simulink model "SCARA"  (R2016a)
settings: Solver=VariableStepAuto  StartTime=0.0  StopTime=10.0  RelTol=1e-3
libraries: powerlib_meascontrol x2, simulink_extras x2
settings Model: Creator=Dominik  LastModifiedBy=Dominik

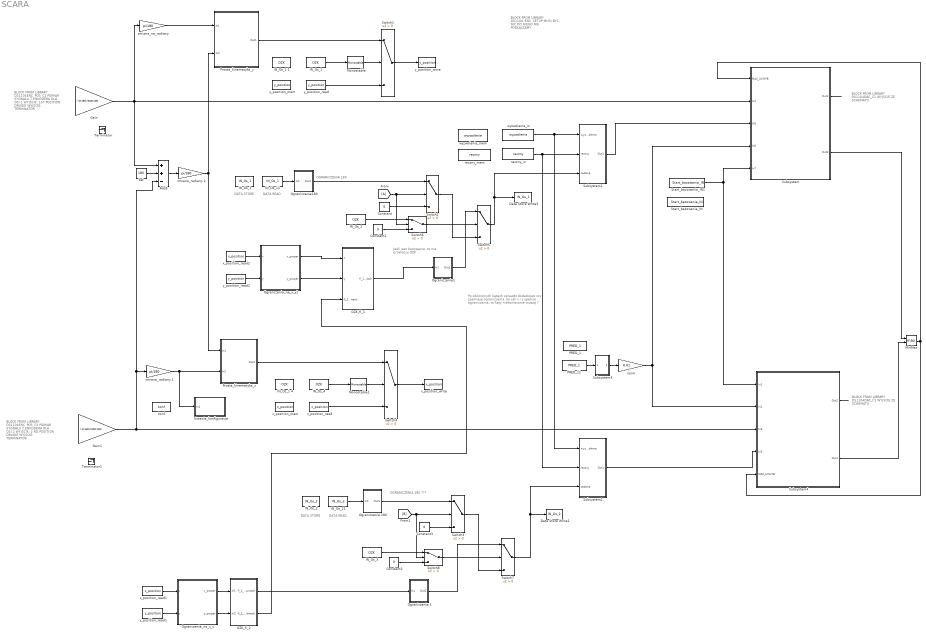
== system SCARA ==
  note: Po obliczonych kątach
      | sprawdź dodatkowo czy spełniają
      | ogranizcenia, bo jak x i y spełnia
      | ograniczenia, to kąty niekoniecznie muszą ?
  note: Jeśli jest bazowanie,
      | to nie przekazuj OZK
  note: DATA READ
  note: DATA STORE
  note: OGRANICZENIA 180
  note: BLOCK FROM LIBRARY
      | DS1104ENC_POS_C1
      | POMIAR SYGNAŁU Z ENKODERA
      | DLA OSI 1
      | WYJŚCIE: 1ST POSITION
      | DRUGIE WYJŚCIE: TERMINATOR
  note: BLOCK FROM LIBRARY
      | DS1104ENC_POS_C2
      | POMIAR SYGNAŁU Z ENKODERA
      | DLA OSI 2
      | WYJŚCIE: 2 ND POSITION
      | DRUGIE WYJŚCIE: TERMINATOR
  note: BLOCK FROM LIBRARY
      | DS1104_ENC_SETUP
      | MUSI BYĆ, NIC DO NIEGO
      | NIE PODŁĄCZAMY
  note: BLOCK FROM LIBRARY
      | DS1104DAC_C1
      | WYJŚCIE ZE SCHEMATU
  note: BLOCK FROM LIBRARY
      | DS1104DAC_C1
      | WYJŚCIE ZE SCHEMATU
  note: OGRANICZENIA 180 ???
  note: DATA STORE
  note: DATA READ
  Add5 : Sum  Inputs=++-
  Constant{,1..3} (4 alike) : Constant  Value=0
  Data Store Write1 : DataStoreWrite  DataStoreName=IN_Os_2
  Data Store Write3 : DataStoreWrite  DataStoreName=IN_Os_1
  Gain : Gain  Gain=(-2*180)/(500*128)
  Gain1 : Gain  Gain=(-2*180)/(500*128)
  IN_Os_{1..4} (4 alike) : DataStoreRead  DataStoreName=OZK
  "IN_Os_1 " : DataStoreMemory  DataStoreName=IN_Os_1  ReadBeforeWriteMsg=warning  WriteAfterWriteMsg=warning  WriteAfterReadMsg=warning  ShowAdditionalParam=off
  IN_Os_1 1 : DataStoreMemory  DataStoreName=OZK  ReadBeforeWriteMsg=warning  WriteAfterWriteMsg=warning  WriteAfterReadMsg=warning  ShowAdditionalParam=off
  IN_Os_1 4 : DataStoreMemory  DataStoreName=OZK  ReadBeforeWriteMsg=warning  WriteAfterWriteMsg=warning  WriteAfterReadMsg=warning  ShowAdditionalParam=off
  IN_Os_11 : DataStoreRead  DataStoreName=IN_Os_1
  "IN_Os_2 " : DataStoreMemory  DataStoreName=IN_Os_2  ReadBeforeWriteMsg=warning  WriteAfterWriteMsg=warning  WriteAfterReadMsg=warning  ShowAdditionalParam=off
  IN_Os_21 : DataStoreRead  DataStoreName=IN_Os_2
  MinMax : MinMax  Function=max  Inputs=2
  Monostable : powerlib_meascontrol/Logic/Monostable  EdgeDetect=Rising  PulseDuration=0.015  ic=0  Ts=0
  Monostable1 : powerlib_meascontrol/Logic/Monostable  EdgeDetect=Rising  PulseDuration=0.015  ic=0  Ts=0
  OZK_fi_1 : Subsystem
  OZK_fi_2 : Subsystem
  Ogranczenia_na_x_y : Subsystem
  Ogranczenia_na_x_y1 : Subsystem
  Ograniczenia 1 : Subsystem
  Ograniczenia 180 : Subsystem
  Ograniczenie1 : Subsystem
  Ograniczenie180 : Subsystem
  "PRED_1 " : DataStoreMemory  DataStoreName=PRED_1  ReadBeforeWriteMsg=warning  WriteAfterWriteMsg=warning  WriteAfterReadMsg=warning  InitialValue=50  ShowAdditionalParam=off
  "PRED_11 " : DataStoreRead  DataStoreName=PRED_1
  Prosta_kinematyka_x : Subsystem
  Prosta_kinematyka_y : Subsystem
  "Start_bazowania_IN " : DataStoreMemory  DataStoreName=Start_bazowania_IN  ReadBeforeWriteMsg=warning  WriteAfterWriteMsg=warning  WriteAfterReadMsg=warning  ShowAdditionalParam=off
  Start_bazowania_IN1 : DataStoreRead  DataStoreName=Start_bazowania_IN
  Subsystem : Subsystem
  Subsystem1 : Subsystem
  Subsystem2 : Subsystem
  Subsystem3 : Subsystem
  Subsystem4 : Subsystem
  Switch{1..8} (8 alike) : Switch  Criteria=u2 > Threshold
  Terminator : Terminator
  Terminator1 : Terminator
  Ustawia_konfiguracje : Subsystem
  "kat " : Constant  Value=180
  konf : DataStoreMemory  DataStoreName=konf  ReadBeforeWriteMsg=warning  WriteAfterWriteMsg=warning  WriteAfterReadMsg=warning  ShowAdditionalParam=off
  norm : Gain  Gain=0.01
  "reczny_in " : DataStoreRead  DataStoreName=reczny
  reczny_mem : DataStoreMemory  DataStoreName=reczny  ReadBeforeWriteMsg=warning  WriteAfterWriteMsg=warning  WriteAfterReadMsg=warning  ShowAdditionalParam=off
  "wyzwolenie_in " : DataStoreRead  DataStoreName=wyzwolenie
  wyzwolenie_mem : DataStoreMemory  DataStoreName=wyzwolenie  ReadBeforeWriteMsg=warning  WriteAfterWriteMsg=warning  WriteAfterReadMsg=warning  ShowAdditionalParam=off
  x_position_mem : DataStoreMemory  DataStoreName=x_position  ReadBeforeWriteMsg=warning  WriteAfterWriteMsg=warning  WriteAfterReadMsg=warning  ShowAdditionalParam=off
  x_position_read : DataStoreRead  DataStoreName=x_position
  x_position_read1 : DataStoreRead  DataStoreName=x_position
  x_position_read2 : DataStoreRead  DataStoreName=x_position
  x_position_write : DataStoreWrite  DataStoreName=x_position
  "y_position_mem " : DataStoreMemory  DataStoreName=y_position  ReadBeforeWriteMsg=warning  WriteAfterWriteMsg=warning  WriteAfterReadMsg=warning  ShowAdditionalParam=off
  y_position_read : DataStoreRead  DataStoreName=y_position
  y_position_read1 : DataStoreRead  DataStoreName=y_position
  y_position_read2 : DataStoreRead  DataStoreName=y_position
  y_position_write : DataStoreWrite  DataStoreName=y_position
  "zmiana_na_radiany " : Gain  Gain=pi/180
  zmiana_radiany 1 : Gain  Gain=pi/180
  zmiana_radiany 2 : Gain  Gain=pi/180
  wires:
  ? -> Gain/1
  ? -> Gain1/1
  ? -> Terminator/1
  ? -> Terminator1/1
  IN_Os_11/1 -> Ograniczenie180/1(In1)
  IN_Os_21/1 -> Ograniczenia 180/1(In1)
  Start_bazowania_IN1/1 -> Subsystem/5(In7), Subsystem4/1(In1)
  Constant/1 -> Switch2/3
  Ograniczenie180/1(Out1) -> Switch2/1
  [A] -> Switch6/2, Switch2/2
  Ograniczenia 180/1(Out1) -> Switch3/1
  Constant3/1 -> Switch3/3
  "wyzwolenie_in "/1 -> Subsystem1/1(wyzwolenie), Subsystem2/1(wyzwolenie)
  "reczny_in "/1 -> Subsystem1/2("reczny "), Subsystem2/2("reczny ")
  "PRED_11 "/1 -> Subsystem3/1(In2)
  norm/1 -> Subsystem4/2(In2), Subsystem/4(In6)
  Subsystem3/1(Out1) -> norm/1
  Subsystem1/1(Out1) -> Subsystem/3(In5)
  Subsystem/1(Out1) -> ?
  Gain1/1 -> Add5/3, zmiana_radiany 1/1, Subsystem4/3(In3)
  Subsystem2/1(Out1) -> Subsystem4/4(In5)
  Subsystem4/1(Out2) -> ?
  Subsystem/2(Out2) -> MinMax/1
  Subsystem4/2(Out1) -> MinMax/2
  MinMax/1 -> Subsystem4/5("MAX_UCHYB "), Subsystem/1("MAX_UCHYB ")
  IN_Os_1/1 -> Monostable/1
  y_position_read/1 -> Switch1/3
  Monostable/1 -> Switch1/2
  Switch1/1 -> y_position_write/1
  IN_Os_4/1 -> Monostable1/1
  x_position_read/1 -> Switch4/3
  Monostable1/1 -> Switch4/2
  Switch4/1 -> x_position_write/1
  "kat "/1 -> Add5/2
  Gain/1 -> "zmiana_na_radiany "/1, Add5/1, Subsystem/2(In2)
  Add5/1 -> zmiana_radiany 2/1
  zmiana_radiany 2/1 -> Prosta_kinematyka_y/2(In2), Prosta_kinematyka_x/1(In1)
  zmiana_radiany 1/1 -> Ustawia_konfiguracje/1(In1), Prosta_kinematyka_x/2(In2)
  Prosta_kinematyka_x/1(Out1) -> Switch4/1
  "zmiana_na_radiany "/1 -> Prosta_kinematyka_y/1(In1)
  Prosta_kinematyka_y/1(Out1) -> Switch1/1
  x_position_read1/1 -> Ogranczenia_na_x_y/1(x)
  y_position_read1/1 -> Ogranczenia_na_x_y/2(y)
  Switch5/1 -> Data Store Write3/1, Subsystem1/3("zadana ")
  Switch2/1 -> Switch5/3
  Ograniczenie1/1(Out1) -> Switch5/1
  IN_Os_2/1 -> Switch6/1
  Constant1/1 -> Switch6/3
  Switch6/1 -> Switch5/2
  x_position_read2/1 -> Ogranczenia_na_x_y1/1(x)
  y_position_read2/1 -> Ogranczenia_na_x_y1/2(y)
  Ogranczenia_na_x_y/1(x_proper) -> OZK_fi_2/1(In1)
  Ogranczenia_na_x_y/2(y_proper) -> OZK_fi_2/2(In2)
  OZK_fi_2/1(fi_2_w_stopniach) -> Ograniczenia 1/1(In1)
  [B] -> Switch8/2, Switch3/2
  IN_Os_3/1 -> Switch8/1
  Constant2/1 -> Switch8/3
  Switch3/1 -> Switch7/3
  Switch8/1 -> Switch7/2
  Ograniczenia 1/1(Out1) -> Switch7/1
  Switch7/1 -> Subsystem2/3("zadana "), Data Store Write1/1
  OZK_fi_2/2(fi_2_w_radianach) -> OZK_fi_1/3(fi_2_w_radianach)
  Ogranczenia_na_x_y1/1(x_proper) -> OZK_fi_1/1(x)
  Ogranczenia_na_x_y1/2(y_proper) -> OZK_fi_1/2(y)
  OZK_fi_1/1(fi_1_w_stopniach) -> Ograniczenie1/1(In1)

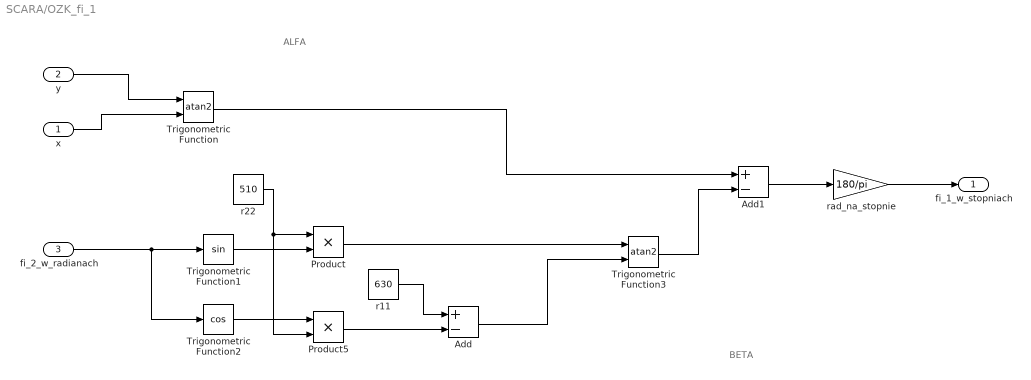
== system SCARA/OZK_fi_1 ==
  note: BETA
  note: ALFA
  x : Inport
  y : Inport  Port=2
  fi_2_w_radianach : Inport  Port=3
  Add : Sum  Inputs=+-
  Add1 : Sum  Inputs=+-
  Product : Product
  Product5 : Product
  Trigonometric Function : Trigonometry  Operator=atan2
  Trigonometric Function1 : Trigonometry
  Trigonometric Function2 : Trigonometry  Operator=cos
  Trigonometric Function3 : Trigonometry  Operator=atan2
  r11 : Constant  Value=630
  r22 : Constant  Value=510
  rad_na_stopnie : Gain  Gain=180/pi
  fi_1_w_stopniach : Outport
  wires:
  fi_2_w_radianach/1 -> Trigonometric Function2/1, Trigonometric Function1/1
  Trigonometric Function1/1 -> Product/2
  r22/1 -> Product5/2, Product/1
  Product/1 -> Trigonometric Function3/1
  Trigonometric Function2/1 -> Product5/1
  r11/1 -> Add/1
  Product5/1 -> Add/2
  Add/1 -> Trigonometric Function3/2
  y/1 -> Trigonometric Function/1
  x/1 -> Trigonometric Function/2
  Trigonometric Function/1 -> Add1/1
  Trigonometric Function3/1 -> Add1/2
  Add1/1 -> rad_na_stopnie/1
  rad_na_stopnie/1 -> fi_1_w_stopniach/1

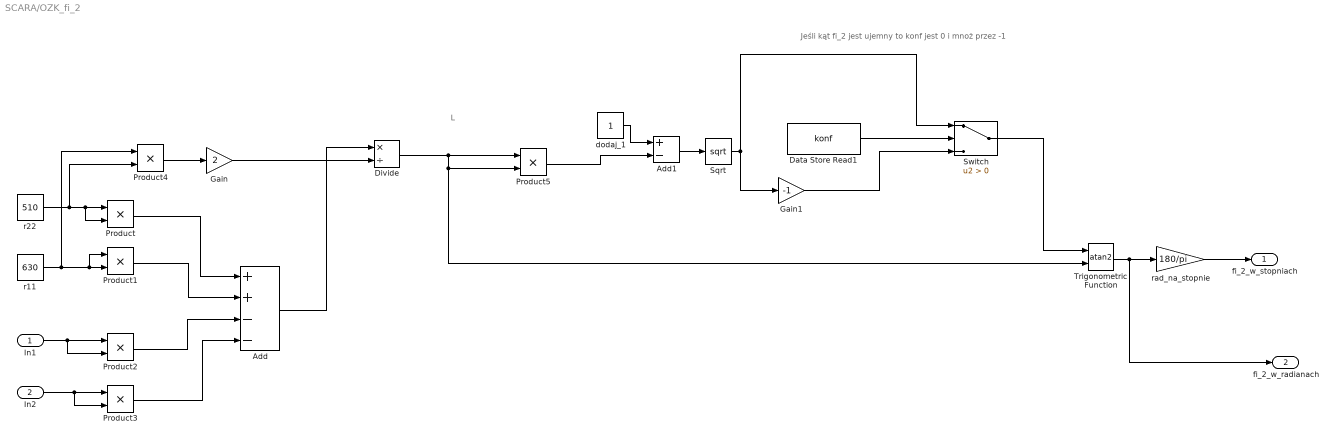
== system SCARA/OZK_fi_2 ==
  note: L
  note: Jeśli kąt fi_2 jest ujemny to konf jest 0
      | i mnoż przez -1
  In1 : Inport
  In2 : Inport  Port=2
  Add : Sum  Inputs=++--
  Add1 : Sum  Inputs=+-
  Data Store Read1 : DataStoreRead  DataStoreName=konf
  Divide : Product  Inputs=*/
  Gain : Gain  Gain=2
  Gain1 : Gain  Gain=-1
  Product{,1..5} (6 alike) : Product
  Sqrt : Sqrt  SaturateOnIntegerOverflow=on
  Switch : Switch  Criteria=u2 > Threshold
  Trigonometric Function : Trigonometry  Operator=atan2
  dodaj_1 : Constant
  r11 : Constant  Value=630
  r22 : Constant  Value=510
  rad_na_stopnie : Gain  Gain=180/pi
  fi_2_w_stopniach : Outport
  fi_2_w_radianach : Outport  Port=2
  wires:
  r22/1 -> Product/2, Product/1, Product4/2
  In1/1 -> Product2/2, Product2/1
  Product1/1 -> Add/2
  Product3/1 -> Add/4
  In2/1 -> Product3/2, Product3/1
  Product/1 -> Add/1
  Product2/1 -> Add/3
  r11/1 -> Product1/1, Product1/2, Product4/1
  Add/1 -> Divide/1
  Product4/1 -> Gain/1
  Gain/1 -> Divide/2
  dodaj_1/1 -> Add1/1
  Add1/1 -> Sqrt/1
  Sqrt/1 -> Gain1/1, Switch/1
  Gain1/1 -> Switch/3
  Switch/1 -> Trigonometric Function/1
  Trigonometric Function/1 -> fi_2_w_radianach/1, rad_na_stopnie/1
  Product5/1 -> Add1/2
  Divide/1 -> Trigonometric Function/2, Product5/2, Product5/1
  Data Store Read1/1 -> Switch/2
  rad_na_stopnie/1 -> fi_2_w_stopniach/1

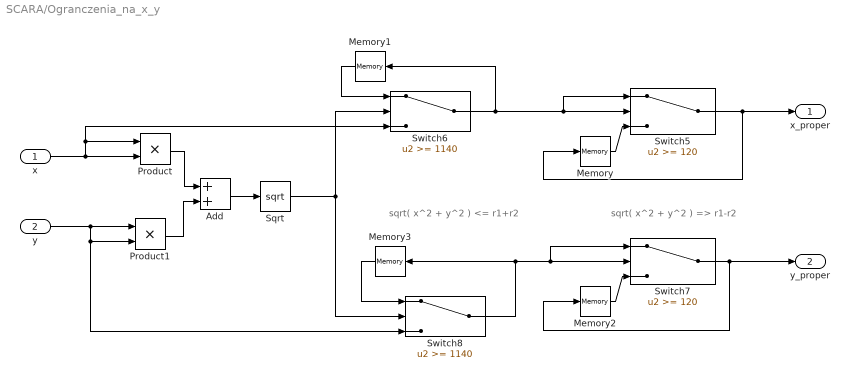
== system SCARA/Ogranczenia_na_x_y ==
  note: sqrt( x^2 + y^2 ) <= r1+r2
  note: sqrt( x^2 + y^2 ) => r1-r2
  x : Inport
  y : Inport  Port=2
  Add : Sum
  Memory{,1..3} (4 alike) : Memory
  Product : Product
  Product1 : Product
  Sqrt : Sqrt  SaturateOnIntegerOverflow=on
  Switch5 : Switch  Threshold=120
  Switch6 : Switch  Threshold=1140
  Switch7 : Switch  Threshold=120
  Switch8 : Switch  Threshold=1140
  x_proper : Outport
  y_proper : Outport  Port=2
  wires:
  Switch5/1 -> x_proper/1, Memory/1
  Switch6/1 -> Switch5/1, Switch5/2, Memory1/1
  Product1/1 -> Add/2
  Memory1/1 -> Switch6/1
  Memory/1 -> Switch5/3
  Switch7/1 -> y_proper/1, Memory2/1
  Memory2/1 -> Switch7/3
  Memory3/1 -> Switch8/1
  Sqrt/1 -> Switch8/2, Switch6/2
  Switch8/1 -> Switch7/1, Switch7/2, Memory3/1
  Add/1 -> Sqrt/1
  y/1 -> Switch8/3, Product1/2, Product1/1
  x/1 -> Product/2, Switch6/3, Product/1
  Product/1 -> Add/1

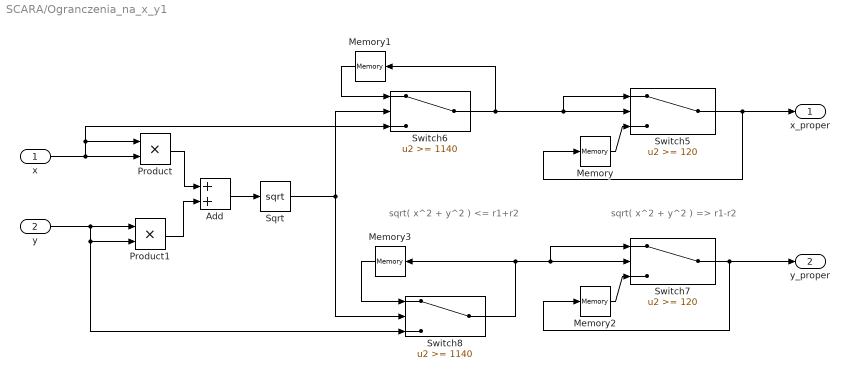
== system SCARA/Ogranczenia_na_x_y1 ==
  note: sqrt( x^2 + y^2 ) <= r1+r2
  note: sqrt( x^2 + y^2 ) => r1-r2
  x : Inport
  y : Inport  Port=2
  Add : Sum
  Memory{,1..3} (4 alike) : Memory
  Product : Product
  Product1 : Product
  Sqrt : Sqrt  SaturateOnIntegerOverflow=on
  Switch5 : Switch  Threshold=120
  Switch6 : Switch  Threshold=1140
  Switch7 : Switch  Threshold=120
  Switch8 : Switch  Threshold=1140
  x_proper : Outport
  y_proper : Outport  Port=2
  wires:
  Switch5/1 -> x_proper/1, Memory/1
  Switch6/1 -> Switch5/1, Switch5/2, Memory1/1
  Product1/1 -> Add/2
  Memory1/1 -> Switch6/1
  Memory/1 -> Switch5/3
  Switch7/1 -> y_proper/1, Memory2/1
  Memory2/1 -> Switch7/3
  Memory3/1 -> Switch8/1
  Sqrt/1 -> Switch8/2, Switch6/2
  Switch8/1 -> Switch7/1, Switch7/2, Memory3/1
  Add/1 -> Sqrt/1
  y/1 -> Switch8/3, Product1/2, Product1/1
  x/1 -> Product/2, Switch6/3, Product/1
  Product/1 -> Add/1

== system SCARA/Ograniczenia 1 ==
  In1 : Inport
  Abs : Abs
  Memory : Memory
  Switch : Switch  Criteria=u2 > Threshold  Threshold=40
  Out1 : Outport
  wires:
  In1/1 -> Switch/3, Abs/1
  Abs/1 -> Switch/2
  Switch/1 -> Memory/1, Out1/1
  Memory/1 -> Switch/1

== system SCARA/Ograniczenia 180 ==
  In1 : Inport
  Abs : Abs
  Memory : Memory
  Switch : Switch  Criteria=u2 > Threshold  Threshold=40
  Out1 : Outport
  wires:
  In1/1 -> Switch/3, Abs/1
  Abs/1 -> Switch/2
  Switch/1 -> Memory/1, Out1/1
  Memory/1 -> Switch/1

== system SCARA/Ograniczenie1 ==
  In1 : Inport
  Abs : Abs
  Memory : Memory
  Switch : Switch  Criteria=u2 > Threshold  Threshold=180
  Out1 : Outport
  wires:
  In1/1 -> Switch/3, Abs/1
  Abs/1 -> Switch/2
  Switch/1 -> Memory/1, Out1/1
  Memory/1 -> Switch/1

== system SCARA/Ograniczenie180 ==
  In1 : Inport
  Abs : Abs
  Memory : Memory
  Switch : Switch  Criteria=u2 > Threshold  Threshold=180
  Out1 : Outport
  wires:
  In1/1 -> Switch/3, Abs/1
  Abs/1 -> Switch/2
  Switch/1 -> Memory/1, Out1/1
  Memory/1 -> Switch/1

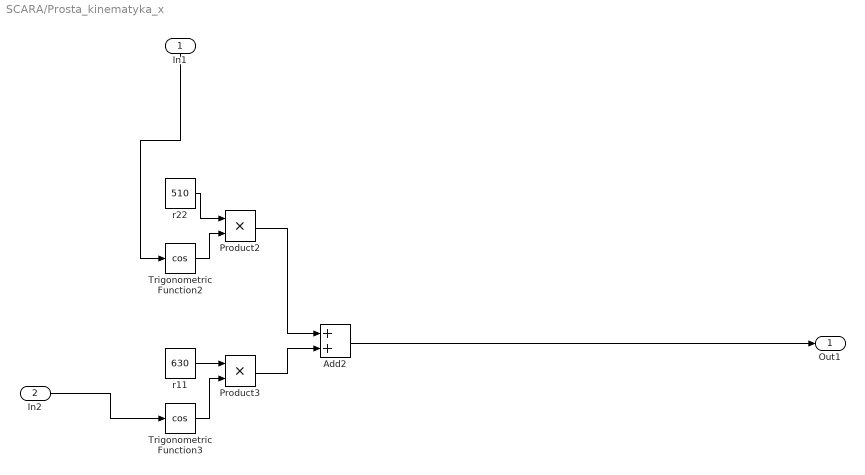
== system SCARA/Prosta_kinematyka_x ==
  In1 : Inport
  In2 : Inport  Port=2
  Add2 : Sum
  Product2 : Product
  Product3 : Product
  Trigonometric Function2 : Trigonometry  Operator=cos
  Trigonometric Function3 : Trigonometry  Operator=cos
  r11 : Constant  Value=630
  r22 : Constant  Value=510
  Out1 : Outport
  wires:
  In2/1 -> Trigonometric Function3/1
  r11/1 -> Product3/1
  r22/1 -> Product2/1
  Add2/1 -> Out1/1
  Trigonometric Function2/1 -> Product2/2
  Trigonometric Function3/1 -> Product3/2
  Product2/1 -> Add2/1
  Product3/1 -> Add2/2
  In1/1 -> Trigonometric Function2/1

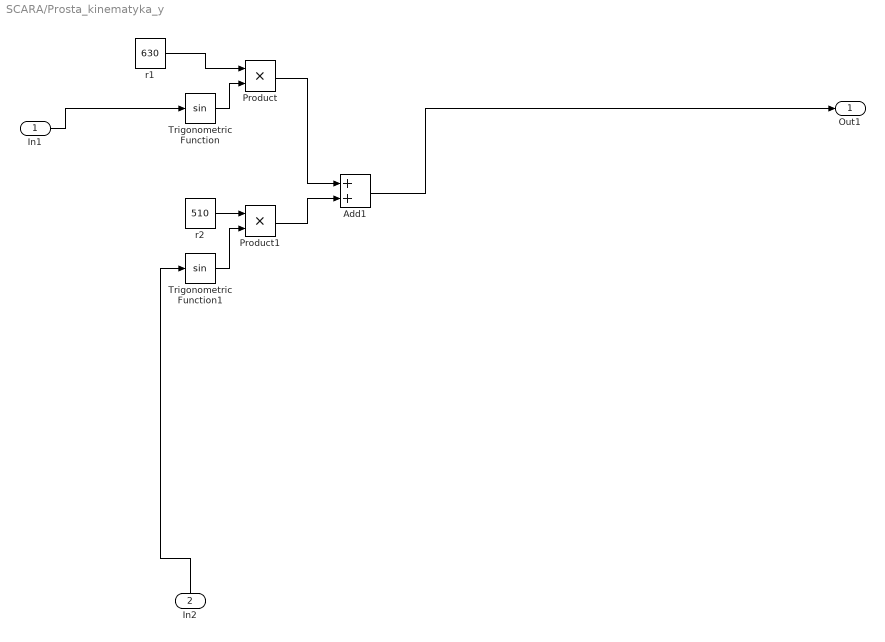
== system SCARA/Prosta_kinematyka_y ==
  In1 : Inport
  In2 : Inport  Port=2
  Add1 : Sum
  Product : Product
  Product1 : Product
  Trigonometric Function : Trigonometry
  Trigonometric Function1 : Trigonometry
  r1 : Constant  Value=630
  r2 : Constant  Value=510
  Out1 : Outport
  wires:
  In1/1 -> Trigonometric Function/1
  Add1/1 -> Out1/1
  r1/1 -> Product/1
  Product/1 -> Add1/1
  Trigonometric Function/1 -> Product/2
  Trigonometric Function1/1 -> Product1/2
  Product1/1 -> Add1/2
  In2/1 -> Trigonometric Function1/1
  r2/1 -> Product1/1

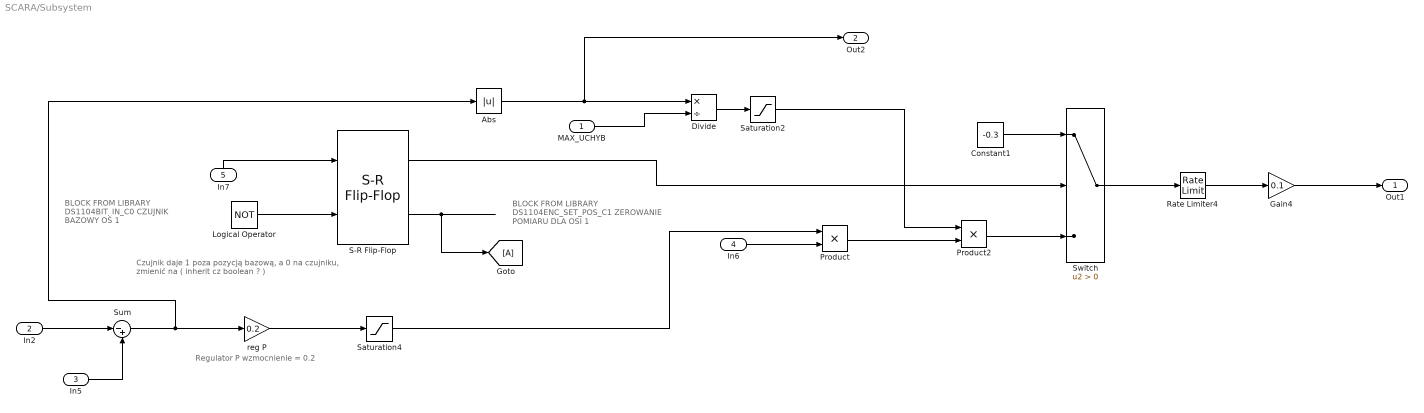
== system SCARA/Subsystem ==
  note: Czujnik daje 1 poza pozycją bazową,
      | a 0 na czujniku, zmienić na ( inherit cz boolean ? )
  note: Regulator P wzmocnienie = 0.2
  note: BLOCK FROM LIBRARY
      | DS1104BIT_IN_C0
      | CZUJNIK BAZOWY OŚ 1
  note: BLOCK FROM LIBRARY
      | DS1104ENC_SET_POS_C1
      | ZEROWANIE POMIARU DLA OSI 1
  "MAX_UCHYB " : Inport
  In2 : Inport  Port=2
  In5 : Inport  Port=3
  In6 : Inport  Port=4
  In7 : Inport  Port=5
  Abs : Abs
  Constant1 : Constant  Value=-0.3
  Divide : Product  Inputs=*/
  Gain4 : Gain  Gain=0.1
  Logical Operator : Logic  Operator=NOT  AllPortsSameDT=off
  Product : Product
  Product2 : Product
  Rate Limiter4 : RateLimiter  RisingSlewLimit=50  FallingSlewLimit=-50  SampleTimeMode=inherited
  S-R Flip-Flop : simulink_extras/Flip Flops/S-R Flip-Flop  initial_condition=0
  Saturation2 : Saturate  UpperLimit=1  LowerLimit=0.001
  Saturation4 : Saturate  UpperLimit=3  LowerLimit=-3
  Sum : Sum  Inputs=|-+
  Switch : Switch  Criteria=u2 > Threshold
  reg P : Gain  Gain=0.2
  Out1 : Outport
  Out2 : Outport  Port=2
  wires:
  Sum/1 -> reg P/1, Abs/1
  Abs/1 -> Out2/1, Divide/1
  "MAX_UCHYB "/1 -> Divide/2
  Divide/1 -> Saturation2/1
  Product/1 -> Product2/2
  Saturation2/1 -> Product2/1
  In7/1 -> S-R Flip-Flop/1
  In6/1 -> Product/2
  In2/1 -> Sum/1
  Rate Limiter4/1 -> Gain4/1
  reg P/1 -> Saturation4/1
  Gain4/1 -> Out1/1
  S-R Flip-Flop/2 -> [A]
  Logical Operator/1 -> S-R Flip-Flop/2
  Switch/1 -> Rate Limiter4/1
  Constant1/1 -> Switch/1
  S-R Flip-Flop/1 -> Switch/2
  ? -> Logical Operator/1
  In5/1 -> Sum/2
  Saturation4/1 -> Product/1
  Product2/1 -> Switch/3

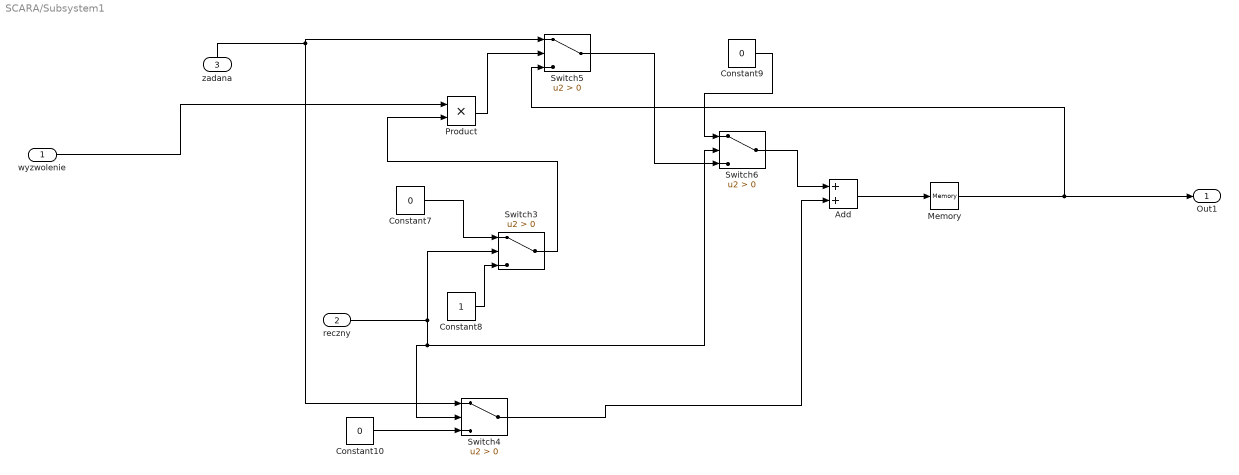
== system SCARA/Subsystem1 ==
  wyzwolenie : Inport
  "reczny " : Inport  Port=2
  "zadana " : Inport  Port=3
  Add : Sum
  Constant10 : Constant  Value=0
  Constant7 : Constant  Value=0
  Constant8 : Constant
  Constant9 : Constant  Value=0
  Memory : Memory
  Product : Product
  Switch{3..6} (4 alike) : Switch  Criteria=u2 > Threshold
  Out1 : Outport
  wires:
  Constant7/1 -> Switch3/1
  Switch4/1 -> Add/2
  "reczny "/1 -> Switch3/2, Switch4/2, Switch6/2
  wyzwolenie/1 -> Product/1
  Add/1 -> Memory/1
  Product/1 -> Switch5/2
  Switch5/1 -> Switch6/3
  "zadana "/1 -> Switch4/1, Switch5/1
  Memory/1 -> Out1/1, Switch5/3
  Constant8/1 -> Switch3/3
  Constant9/1 -> Switch6/1
  Constant10/1 -> Switch4/3
  Switch3/1 -> Product/2
  Switch6/1 -> Add/1

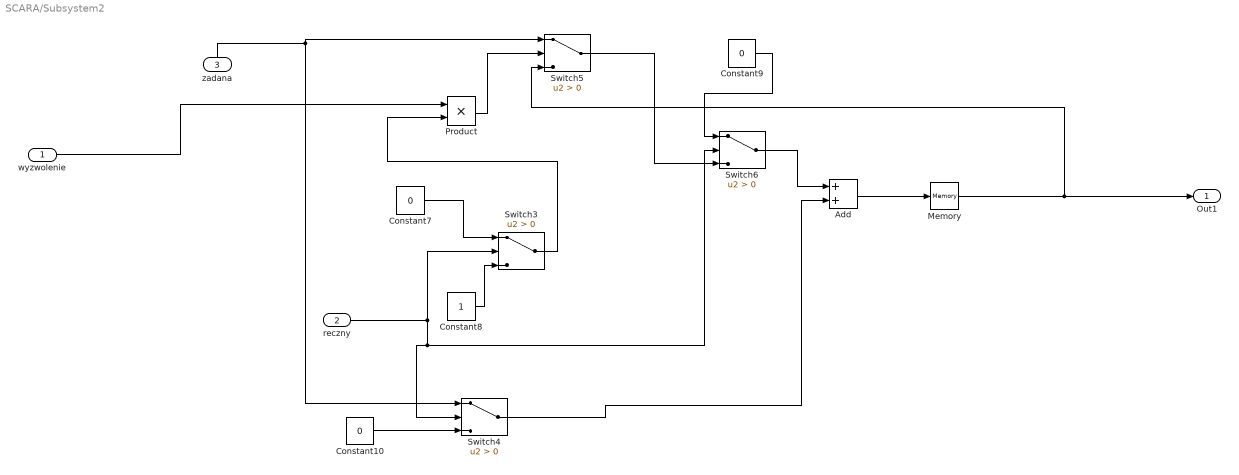
== system SCARA/Subsystem2 ==
  wyzwolenie : Inport
  "reczny " : Inport  Port=2
  "zadana " : Inport  Port=3
  Add : Sum
  Constant10 : Constant  Value=0
  Constant7 : Constant  Value=0
  Constant8 : Constant
  Constant9 : Constant  Value=0
  Memory : Memory
  Product : Product
  Switch{3..6} (4 alike) : Switch  Criteria=u2 > Threshold
  Out1 : Outport
  wires:
  Constant7/1 -> Switch3/1
  Switch4/1 -> Add/2
  "reczny "/1 -> Switch3/2, Switch4/2, Switch6/2
  wyzwolenie/1 -> Product/1
  Add/1 -> Memory/1
  Product/1 -> Switch5/2
  Switch5/1 -> Switch6/3
  "zadana "/1 -> Switch4/1, Switch5/1
  Memory/1 -> Out1/1, Switch5/3
  Constant8/1 -> Switch3/3
  Constant9/1 -> Switch6/1
  Constant10/1 -> Switch4/3
  Switch3/1 -> Product/2
  Switch6/1 -> Add/1

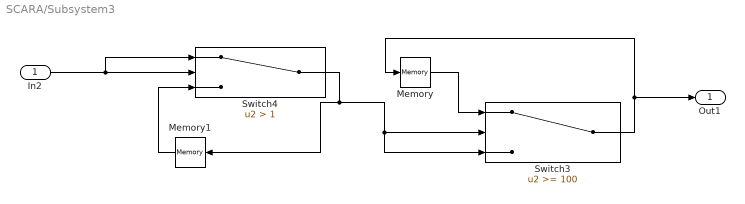
== system SCARA/Subsystem3 ==
  In2 : Inport
  Memory : Memory
  Memory1 : Memory
  Switch3 : Switch  Threshold=100
  Switch4 : Switch  Criteria=u2 > Threshold  Threshold=1
  Out1 : Outport
  wires:
  Switch4/1 -> Memory1/1, Switch3/3, Switch3/2
  Memory1/1 -> Switch4/3
  Switch3/1 -> Memory/1, Out1/1
  In2/1 -> Switch4/1, Switch4/2
  Memory/1 -> Switch3/1

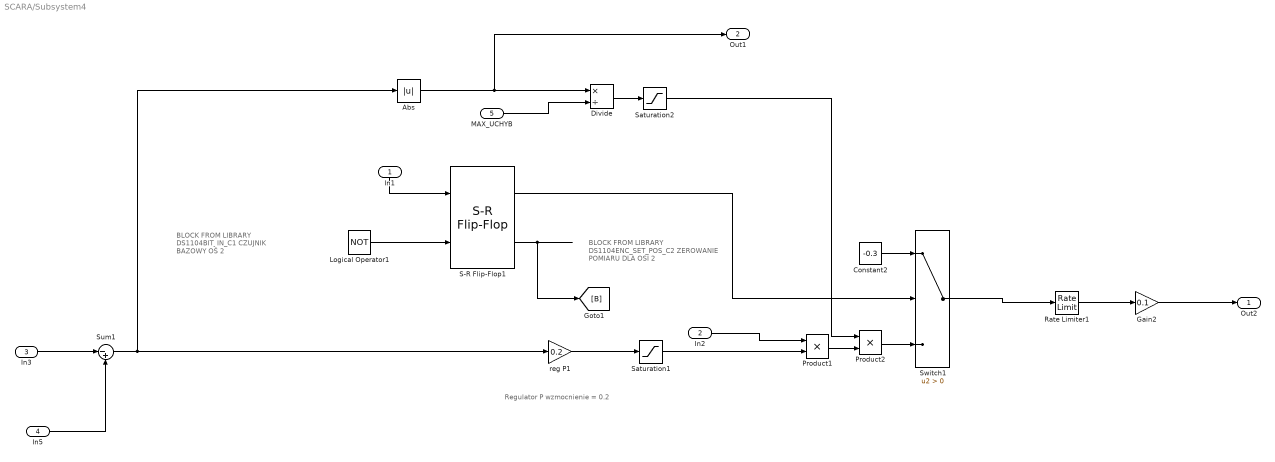
== system SCARA/Subsystem4 ==
  note: Regulator P wzmocnienie = 0.2
  note: BLOCK FROM LIBRARY
      | DS1104BIT_IN_C1
      | CZUJNIK BAZOWY OŚ 2
  note: BLOCK FROM LIBRARY
      | DS1104ENC_SET_POS_C2
      | ZEROWANIE POMIARU DLA OSI 2
  In1 : Inport
  In2 : Inport  Port=2
  In3 : Inport  Port=3
  In5 : Inport  Port=4
  "MAX_UCHYB " : Inport  Port=5
  Abs : Abs
  Constant2 : Constant  Value=-0.3
  Divide : Product  Inputs=*/
  Gain2 : Gain  Gain=0.1
  Logical Operator1 : Logic  Operator=NOT  AllPortsSameDT=off
  Product1 : Product
  Product2 : Product
  Rate Limiter1 : RateLimiter  RisingSlewLimit=50  FallingSlewLimit=-50  SampleTimeMode=inherited
  S-R Flip-Flop1 : simulink_extras/Flip Flops/S-R Flip-Flop  initial_condition=0
  Saturation1 : Saturate  UpperLimit=3  LowerLimit=-3
  Saturation2 : Saturate  UpperLimit=1  LowerLimit=0.001
  Sum1 : Sum  Inputs=|-+
  Switch1 : Switch  Criteria=u2 > Threshold
  reg P1 : Gain  Gain=0.2
  Out2 : Outport
  Out1 : Outport  Port=2
  wires:
  In2/1 -> Product1/1
  In1/1 -> S-R Flip-Flop1/1
  In3/1 -> Sum1/1
  Sum1/1 -> Abs/1, reg P1/1
  Rate Limiter1/1 -> Gain2/1
  Gain2/1 -> Out2/1
  reg P1/1 -> Saturation1/1
  Switch1/1 -> Rate Limiter1/1
  Constant2/1 -> Switch1/1
  S-R Flip-Flop1/1 -> Switch1/2
  In5/1 -> Sum1/2
  ? -> Logical Operator1/1
  Logical Operator1/1 -> S-R Flip-Flop1/2
  S-R Flip-Flop1/2 -> [B]
  Saturation1/1 -> Product1/2
  Abs/1 -> Out1/1, Divide/1
  "MAX_UCHYB "/1 -> Divide/2
  Divide/1 -> Saturation2/1
  Saturation2/1 -> Product2/1
  Product1/1 -> Product2/2
  Product2/1 -> Switch1/3

== system SCARA/Ustawia_konfiguracje ==
  note: Jeśli fi_2 większe od 0, to 1, a jak nie to 0
  In1 : Inport
  Constant2 : Constant
  Constant4 : Constant  Value=0
  Data Store Write : DataStoreWrite  DataStoreName=konf
  Switch : Switch  Criteria=u2 > Threshold
  wires:
  In1/1 -> Switch/2
  Switch/1 -> Data Store Write/1
  Constant2/1 -> Switch/1
  Constant4/1 -> Switch/3
